simulink model "Hopper_1DOF"  (R2025a)
settings: Solver=VariableStepAuto  StartTime=0.0  StopTime=50  RelTol=1e-3
values from neighbouring files (symbols this model uses):
  bp = data(:,1)    [load_lookup.m]
  IN =     [hopper_sizing_output.mat]    (also in main.m = mission_inputs())
  OUT =     [hopper_sizing_output.mat]    (also in main.m = Outputs(IN, VEH, TANKS, STRUCT))
undefined symbols (not defined in the file or in its folder): tbl1, tbl2
libraries: SignalEditorBlockLib x1
settings Model: Creator=asing  LastModifiedBy=asing

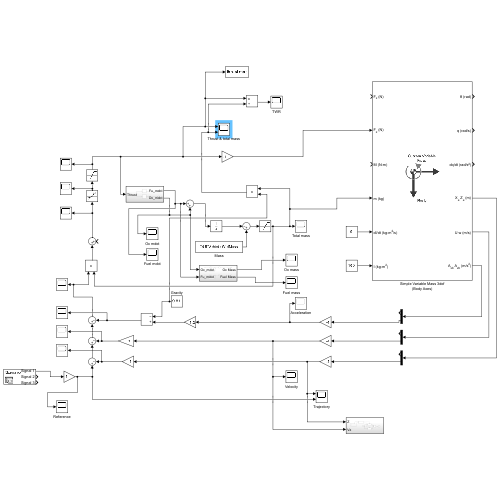
[thumbnail: Simulink's stored preview of the top-level diagram]
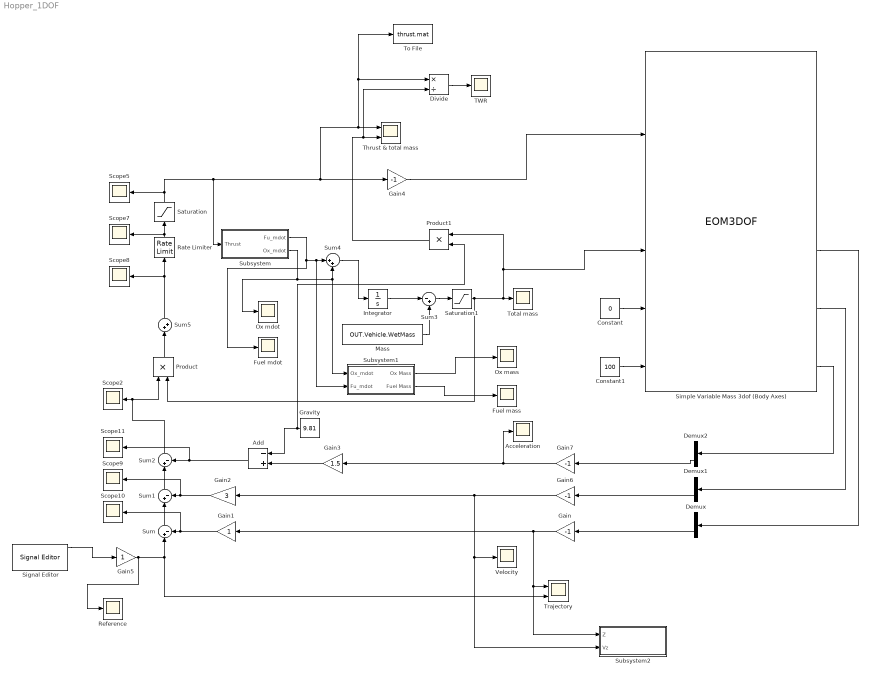
== system Hopper_1DOF ==
  Acceleration : Scope
      settings: ActiveDisplayYMinimum=-1.9767019185311641  ActiveDisplayYMaximum=2.7900822902807079  DataLoggingVariableName=ScopeData3
  Add : Sum  Inputs=-+
  Constant : Constant  Value=0
  Constant1 : Constant  Value=100
  Demux : Demux  Outputs=2
  Demux1 : Demux  Outputs=2
  Demux2 : Demux  Outputs=2
  Divide : Product  Inputs=*/
  Fuel mass : Scope
      settings: ActiveDisplayYMinimum=3.3852654059846028  ActiveDisplayYMaximum=9.6238593993350445  DataLoggingVariableName=ScopeData13
  Fuel mdot : Scope
      settings: ActiveDisplayYMinimum=-1  ActiveDisplayYMaximum=1  DataLoggingVariableName=ScopeData16
  Gain{,4,6..7} (4 alike) : Gain  Gain=-1
  Gain1 : Gain
  Gain2 : Gain  Gain=3
  Gain3 : Gain  Gain=1.5
  Gain5 : Gain
  Gravity : Constant  Value=9.81
  Integrator : Integrator
  Mass : Constant  Value=OUT.Vehicle.WetMass
  Ox mass : Scope
      settings: ActiveDisplayYMinimum=-1  ActiveDisplayYMaximum=1  DataLoggingVariableName=ScopeData6
  Ox mdot : Scope
      settings: ActiveDisplayYMinimum=-1  ActiveDisplayYMaximum=1  DataLoggingVariableName=ScopeData15
  Product : Product
  Product1 : Product
  Rate Limiter : RateLimiter  RisingSlewLimit=800  FallingSlewLimit=-800  SampleTimeMode=inherited
  Reference : Scope
      settings: ActiveDisplayYMinimum=-1  ActiveDisplayYMaximum=1  DataLoggingVariableName=ScopeData14
  Saturation : Saturate  UpperLimit=2400  LowerLimit=890  ZeroCross=off
  Saturation1 : Saturate  UpperLimit=OUT.Vehicle.WetMass  LowerLimit=OUT.Vehicle.DryMass
  Scope{2,5,7..11} (7 alike) : Scope
      Scope10 settings: ActiveDisplayYMinimum=2.5668663178756459  ActiveDisplayYMaximum=5.1587087678696406  DataLoggingVariableName=ScopeData10
      Scope11 settings: ActiveDisplayYMinimum=-12.678408094760533  ActiveDisplayYMaximum=11.36813163204156  DataLoggingVariableName=ScopeData11
      Scope2 settings: ActiveDisplayYMinimum=-1.2963468600802761  ActiveDisplayYMaximum=12.866662972523486  DataLoggingVariableName=ScopeData2
      Scope5 settings: ActiveDisplayYMinimum=262.50000000000006  ActiveDisplayYMaximum=2637.5  DataLoggingVariableName=ScopeData5
      Scope7 settings: ActiveDisplayYMinimum=-867.34301243195137  ActiveDisplayYMaximum=3667.8043798582971  DataLoggingVariableName=ScopeData7
      Scope8 settings: ActiveDisplayYMinimum=-820.83409646301129  ActiveDisplayYMaximum=1825.4371218292233  DataLoggingVariableName=ScopeData8
      Scope9 settings: ActiveDisplayYMinimum=-1  ActiveDisplayYMaximum=1  DataLoggingVariableName=ScopeData9
  Signal Editor : SignalEditorBlockLib/Signal Editor  FileName=trajectory_1.mat  ActiveScenario=Scenario  ActiveSignal=Signal 3  IsBus=off  OutputBusObjectStr=Bus: BusObject  SampleTime=0  ZeroCross=off  OutputAfterFinalValue=Setting to zero  Unit=inherit  PreserveSignalName=on  ApplySigPropsToAllScenarios=on  ApplySigPropsToAllSignals=off  SignalPropertySource=Dialog parameters
  Simple Variable Mass 3dof (Body Axes) : EOM3DOF  mtype=Custom Variable  v_ini=0  mass=100  mass_e=50  mass_f=100  Iyy_e=2500  Iyy_f=5000
  Subsystem : Subsystem
  Subsystem1 : Subsystem
  Subsystem2 : Subsystem
  Sum : Sum  Inputs=|+-
  Sum1 : Sum  Inputs=|+-
  Sum2 : Sum  Inputs=|+-
  Sum3 : Sum  Inputs=|-+
  Sum4 : Sum  Inputs=|++
  Sum5 : Sum  Inputs=|++
  TWR : Scope
      settings: ActiveDisplayYMinimum=-1  ActiveDisplayYMaximum=1  DataLoggingVariableName=ScopeData17
  Thrust & total mass : Scope  NumInputPorts=2
      settings: ActiveDisplayYMinimum=834.82891041187213  ActiveDisplayYMaximum=1386.5398062931506
  To File : ToFile  Filename=thrust.mat  SaveFormat=Timeseries
  Total mass : Scope
      settings: ActiveDisplayYMinimum=104.08322056806487  ActiveDisplayYMaximum=121.9933343110873  DataLoggingVariableName=ScopeData4
  Trajectory : Scope  NumInputPorts=2
      settings: ActiveDisplayYMinimum=-6.39214076445119  ActiveDisplayYMaximum=57.529266880060725
  Velocity : Scope
      settings: ActiveDisplayYMinimum=-9.0313628520240385  ActiveDisplayYMaximum=10.233384680482745  DataLoggingVariableName=ScopeData12
  wires:
  Simple Variable Mass 3dof (Body Axes)/4 -> Demux/1
  Demux/2 -> Gain/1
  Gain/1 -> Subsystem2/1(Z), Trajectory/1, Gain1/1
  Sum/1 -> Sum1/1
  Sum1/1 -> Sum2/1
  Gain1/1 -> Scope10/1, Sum/2
  Simple Variable Mass 3dof (Body Axes)/5 -> Demux1/1
  Simple Variable Mass 3dof (Body Axes)/6 -> Demux2/1
  Demux1/2 -> Gain6/1
  Gain2/1 -> Scope9/1, Sum1/2
  Gain4/1 -> Simple Variable Mass 3dof (Body Axes)/2
  Rate Limiter/1 -> Saturation/1, Scope7/1
  Demux2/2 -> Gain7/1
  Sum4/1 -> Integrator/1
  Integrator/1 -> Sum3/1
  Sum3/1 -> Saturation1/1
  Mass/1 -> Sum3/2
  Sum2/1 -> Product/1, Scope2/1
  Saturation/1 -> Scope5/1, Subsystem/1(Thrust), Gain4/1, Divide/1, To File/1, Thrust & total mass/1
  Gain6/1 -> Subsystem2/2(Vz), Velocity/1, Gain2/1
  Gain7/1 -> Acceleration/1, Gain3/1
  Gain3/1 -> Add/2
  Add/1 -> Scope11/1, Sum2/2
  Constant/1 -> Simple Variable Mass 3dof (Body Axes)/5
  Constant1/1 -> Simple Variable Mass 3dof (Body Axes)/6
  Gravity/1 -> Product1/2, Add/1
  Subsystem/1(Fu_mdot) -> Fuel mdot/1, Subsystem1/2(Fu_mdot), Sum4/1
  Subsystem/2(Ox_mdot) -> Ox mdot/1, Subsystem1/1(Ox_mdot), Sum4/2
  Subsystem1/1(Ox Mass) -> Ox mass/1
  Subsystem1/2(Fuel Mass) -> Fuel mass/1
  Gain5/1 -> Reference/1, Trajectory/2, Sum/1
  Sum5/1 -> Scope8/1, Rate Limiter/1
  Saturation1/1 -> Product/2, Product1/1, Simple Variable Mass 3dof (Body Axes)/4, Total mass/1
  Signal Editor/1 -> Gain5/1
  Product/1 -> Sum5/1
  Product1/1 -> Divide/2, Thrust & total mass/2
  Divide/1 -> TWR/1

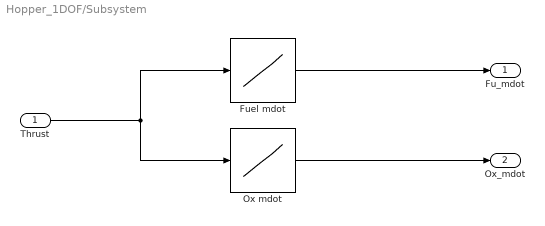
== system Hopper_1DOF/Subsystem ==
  Thrust : Inport
  Fuel mdot : Lookup_n-D  NumberOfTableDimensions=1  BreakpointsForDimension1=bp  Table=tbl2  InternalRulePriority=Speed  RndMeth=Simplest
  Ox mdot : Lookup_n-D  NumberOfTableDimensions=1  BreakpointsForDimension1=bp  Table=tbl1  InternalRulePriority=Speed  RndMeth=Simplest
  Fu_mdot : Outport
  Ox_mdot : Outport  Port=2
  wires:
  Thrust/1 -> Ox mdot/1, Fuel mdot/1
  Fuel mdot/1 -> Fu_mdot/1
  Ox mdot/1 -> Ox_mdot/1

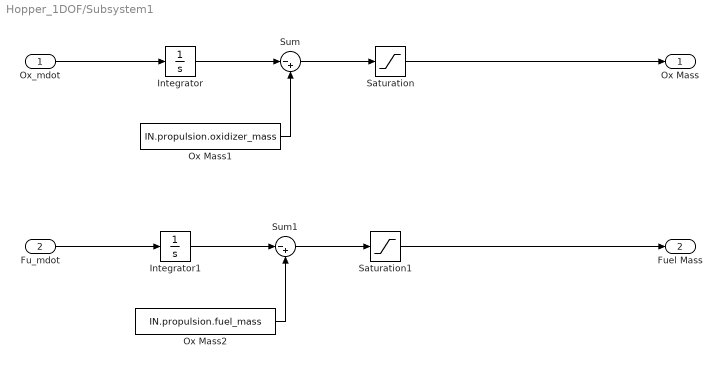
== system Hopper_1DOF/Subsystem1 ==
  Ox_mdot : Inport
  Fu_mdot : Inport  Port=2
  Integrator : Integrator
  Integrator1 : Integrator
  Ox Mass1 : Constant  Value=IN.propulsion.oxidizer_mass
  Ox Mass2 : Constant  Value=IN.propulsion.fuel_mass
  Saturation : Saturate  UpperLimit=IN.propulsion.oxidizer_mass  LowerLimit=0
  Saturation1 : Saturate  UpperLimit=IN.propulsion.fuel_mass  LowerLimit=0
  Sum : Sum  Inputs=|-+
  Sum1 : Sum  Inputs=|-+
  Ox Mass : Outport
  Fuel Mass : Outport  Port=2
  wires:
  Ox_mdot/1 -> Integrator/1
  Integrator/1 -> Sum/1
  Ox Mass1/1 -> Sum/2
  Sum/1 -> Saturation/1
  Saturation/1 -> Ox Mass/1
  Sum1/1 -> Saturation1/1
  Saturation1/1 -> Fuel Mass/1
  Fu_mdot/1 -> Integrator1/1
  Ox Mass2/1 -> Sum1/2
  Integrator1/1 -> Sum1/1

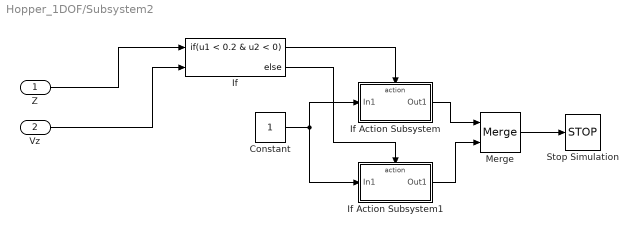
== system Hopper_1DOF/Subsystem2 ==
  Z : Inport
  Vz : Inport  Port=2
  Constant : Constant
  If : If  NumInputs=2  IfExpression=u1 < 0.2 & u2 < 0
  If Action Subsystem : Subsystem  TreatAsAtomicUnit=on
  If Action Subsystem1 : Subsystem  TreatAsAtomicUnit=on
  Merge : Merge
  Stop Simulation : Stop
  wires:
  Z/1 -> If/1
  Vz/1 -> If/2
  If/1 -> If Action Subsystem/Action
  If/2 -> If Action Subsystem1/Action
  Constant/1 -> If Action Subsystem1/1(In1), If Action Subsystem/1(In1)
  If Action Subsystem/1(Out1) -> Merge/1
  If Action Subsystem1/1(Out1) -> Merge/2
  Merge/1 -> Stop Simulation/1

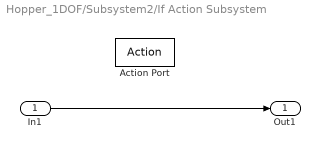
== system Hopper_1DOF/Subsystem2/If Action Subsystem ==
  In1 : Inport
  Action Port : ActionPort  ActionPortLabel=if(u1 < 0.2 & u2 < 0)
  Out1 : Outport
  wires:
  In1/1 -> Out1/1

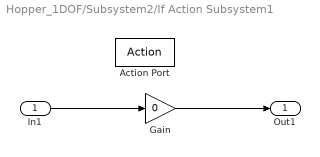
== system Hopper_1DOF/Subsystem2/If Action Subsystem1 ==
  In1 : Inport
  Action Port : ActionPort  ActionPortLabel=else
  Gain : Gain  Gain=0
  Out1 : Outport
  wires:
  In1/1 -> Gain/1
  Gain/1 -> Out1/1
